simulink model "P1"  (R2018a)
settings: Solver=VariableStepAuto  StartTime=0.0  StopTime=300  RelTol=1e-3
undefined symbols (not defined in the file or in its folder): m, n
settings Model: Creator=aminrakhsha  LastModifiedBy=whitefox

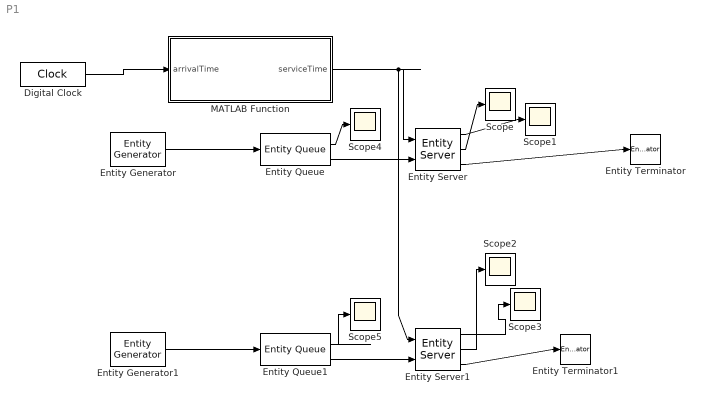
== system P1 ==
  Digital Clock : DigitalClock  SampleTime=1000
  Entity Generator : EntityGenerator  OutputPortMessageModes=m  TimeSource=MATLAB action  Period=5  IntergenerationTimeAction=|  EntityType=Structured  EntityTypeName=Entity
      | mean=2;
      | dt = -mean*log(1-rand());
  Entity Generator1 : EntityGenerator  OutputPortMessageModes=m  TimeSource=MATLAB action  IntergenerationTimeAction=|  EntityType=Structured  EntityTypeName=Entity
      | mean=2;
      | dt = -mean*log(1-rand());
  Entity Queue : EntityQueue  InputPortMessageModes=m  OutputPortMessageModes=n,m  Capacity=inf  AverageWait=on
      settings: OutputPortMap=o2,o5
  Entity Queue1 : EntityQueue  InputPortMessageModes=m  OutputPortMessageModes=n,m  Capacity=inf  QueueType=LIFO  AverageWait=on
      settings: OutputPortMap=o2,o5
  Entity Server : EntityServer  InputPortMessageModes=n,m  OutputPortMessageModes=n,n,m  Capacity=1  ServiceTimeSource=Signal port  ServiceTimeAttributeName=Attribute1  ServiceTimeAction=dt = getST(y);  AverageWait=on  Utilization=on
      settings: InputPortMap=u0,u2  OutputPortMap=o4,o5,o9
  Entity Server1 : EntityServer  InputPortMessageModes=n,m  OutputPortMessageModes=n,n,m  Capacity=1  ServiceTimeSource=Signal port  AverageWait=on  Utilization=on
      settings: InputPortMap=u0,u2  OutputPortMap=o4,o5,o9
  Entity Terminator : EntityTerminator  InputPortMessageModes=m
  Entity Terminator1 : EntityTerminator  InputPortMessageModes=m
  MATLAB Function : MATLAB Function  TreatAsAtomicUnit=on
  Scope{,1..5} (6 alike) : Scope
  wires:
  Entity Generator/1 -> Entity Queue/1
  Entity Queue/2 -> Entity Server/2
  Entity Server/3 -> Entity Terminator/1
  Entity Generator1/1 -> Entity Queue1/1
  Entity Queue1/2 -> Entity Server1/2
  Entity Server1/3 -> Entity Terminator1/1
  Entity Server/2 -> Scope/1
  Entity Server/1 -> Scope1/1
  Digital Clock/1 -> MATLAB Function/1(arrivalTime)
  Entity Server1/2 -> Scope2/1
  Entity Server1/1 -> Scope3/1
  Entity Queue1/1 -> Scope5/1
  Entity Queue/1 -> Scope4/1
  MATLAB Function/1(serviceTime) -> Entity Server/1, Entity Server1/1

== matlab function P1/MATLAB Function ==
  data: arrivalTime input; serviceTime output
% consider the case in which our servers are humans and by passing time
% they become tired and their servicetimes increases 
function serviceTime = serviceTimeFunction(arrivalTime)
    mean = 0;
    if arrivalTime < 100
        mean = 1;
    elseif arrivalTime >= 100 && arrivalTime < 200
        mean = 2;
    elseif arrivalTime >= 200 && arrivalTime < 300
        mean = 4;
    elseif arrivalTime >= 300 && arrivalTime < 400
        mean = 8;
    else
        mean = 16;
    end   
    serviceTime = -mean*log(1-rand());
%     serviceTime = mean
